simulink model "Demo_MinSegNano_V3_20b"  (R2020b)
settings: Solver=FixedStepDiscrete  StartTime=0.0  StopTime=inf  FixedStep=.03  RelTol=1e-3  EnableMultiTasking=on
undefined symbols (not defined in the file): TS
libraries: arduinolib x6, RASPlib x6, MinSegLibrary_MinSegNano x4, svdutilitieslib x4
settings Model: SILPILModeSetting=veronly  ExtModeTrigDuration=2  Creator=Alec  LastModifiedBy=hurstj
settings DataIOCC: LimitDataPoints=on  SaveFormat=Array  ReturnWorkspaceOutputs=off
settings OptimizationCC: EnhancedBackFolding=on  PassReuseOutputArgsAs=Individual arguments  ExpressionDepthLimit=2147483647  ZeroExternalMemoryAtStartup=off  ZeroInternalMemoryAtStartup=off  MaxStackSize=64  OptimizeBlockOrder=speed  DifferentSizesBufferReuse=on  OptimizationCustomize=off  EfficientTunableParamExpr=on
settings DebuggingCC: UnderspecifiedInitializationDetection=Classic  MergeDetectMultiDrivingBlocksExec=none  ParameterTunabilityLossMsg=error  StateNameClashWarn=warning  SFUnexpectedBacktrackingDiag=warning  SFNoUnconditionalDefaultTransitionDiag=warning  SFExecutionAtInitializationDiag=none  ArithmeticOperatorsInVariantConditions=warning
settings HardwareCC: ProdBitPerInt=16  ProdBitPerPointer=16  ProdBitPerSizeT=16  ProdBitPerPtrDiffT=16  ProdLargestAtomicFloat=None  ProdWordSize=8  ProdHWDeviceType=Atmel->AVR  UseEmbeddedCoderFeatures=off  UseSimulinkCoderFeatures=off
settings ModelReferenceCC: PropagateSignalLabelsOutOfModel=off
settings SFSimCC: SimUseLocalCustomCode=off  MATLABDynamicMemAlloc=off  CustomCodeUndefinedFunction=UseInterfaceOnly
settings RTWCC: Description=Embedded Coder  SystemTargetFile=ert.tlc  HardwareBoard=Arduino Nano 3.0  TemplateMakefile=ert_default_tmf  RTWVerbose=off  RTWUseLocalCustomCode=off  Toolchain=Arduino AVR  BuildConfiguration=Faster Runs
settings CodeAppCC: ForceParamTrailComments=on  IgnoreCustomStorageClasses=off  OperatorAnnotations=on  SimulinkDataObjDesc=on  SFDataObjDesc=on  CustomSymbolStrType=$N$R$M  InsertBlockDesc=on  InternalIdentifier=Classic
settings ERTTargetCC: SupportContinuousTime=on  SupportNonInlinedSFcns=on  SupportVariableSizeSignals=on  ExtModeStaticAllocSize=250
settings ConfigComp: CovMetricSettings=dw  CovSaveCumulativeToWorkspaceVar=on  CovSaveSingleToWorkspaceVar=on  CovExternalEMLEnable=off

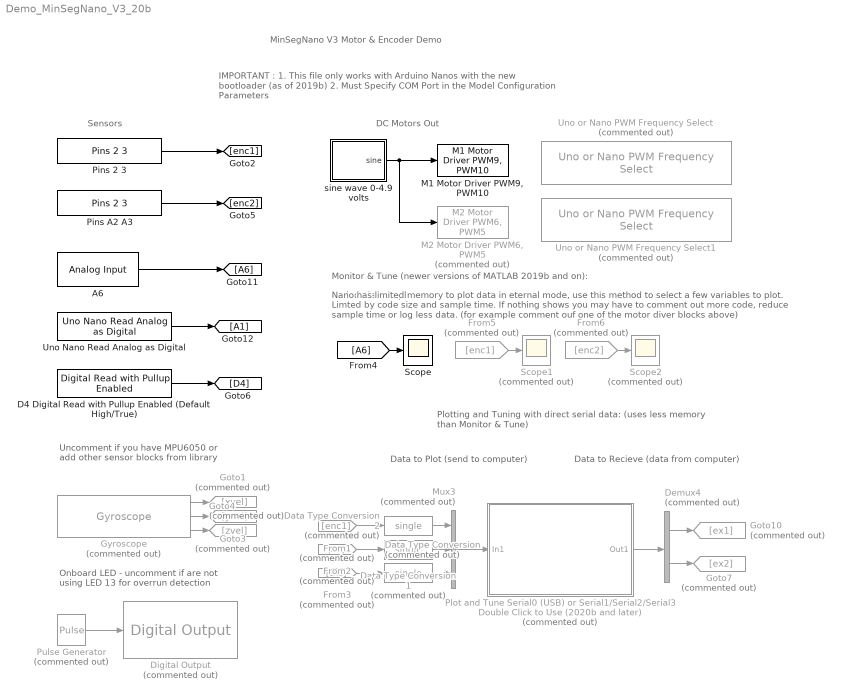
== system Demo_MinSegNano_V3_20b ==
  note: Onboard LED - uncomment if are not
      | using LED 13 for overrun detection
  note: Uncomment if you have MPU6050 or
      | add other sensor blocks from library
  note: Plotting and Tuning with direct serial data:
      | (uses less memory than Monitor & Tune)
  note: DC Motors Out
  note: Sensors
  note: MinSegNano V3 Motor & Encoder Demo
  note: IMPORTANT :
      | 1. This file only works with Arduino Nanos with the new bootloader (as of 2019b)
      | 2. Must Specify COM Port in the Model Configuration Parameters
  note: Monitor & Tune (newer versions of MATLAB 2019b and on):
  note: select data to plot
  note: Nano has limited memory to plot data in eternal mode, use this method to select a few variables to plot. Limted by code size and sample time. If nothing shows you may have to comment out more code, reduce sample time or log less data. (for example comment ouf one of the motor diver blocks above)
  note: Data to Plot
      | (send to computer)
  note: Data to Recieve
      | (data from computer)
  A6 : arduinolib/Analog Input  pinNumber=6  ReadResultsOnly=off  ConversionTriggerSource=Software  ExternalTriggerType=uint32( 0 )  OutputDataType=uint16  EnableConversionCompleteNotify=off  EnableOuputStatus=off  SampleTime=-1  blockPlatform=arduino
  D4 Digital Read with Pullup Enabled (Default High/True) : RASPlib/Digital Read with Pullup Enabled  Pin=4
      settings: SourceProductName=Rensselaer Arduino Support Package
  Data Type Conversion : DataTypeConversion  Commented=on  OutDataTypeStr=single
  Data Type Conversion1 : DataTypeConversion  Commented=on  OutDataTypeStr=single
  Data Type Conversion2 : DataTypeConversion  Commented=on  OutDataTypeStr=single
  Demux4 : Demux  Commented=on  Outputs=2
  Digital Output : arduinolib/Digital Output  Commented=on  pinNumber=13  Direction=output  blockPlatform=arduino
  From1 : From  Commented=on  GotoTag=enc1
  From2 : From  Commented=on  GotoTag=A6
  From3 : From  Commented=on  GotoTag=ex1
  From5 : From  Commented=on  GotoTag=enc1
  From6 : From  Commented=on  GotoTag=enc2
  Goto1 : Goto  Commented=on  GotoTag=xvel
  Goto10 : Goto  Commented=on  GotoTag=ex1
  Goto3 : Goto  Commented=on  GotoTag=yvel
  Goto4 : Goto  Commented=on  GotoTag=zvel
  Goto7 : Goto  Commented=on  GotoTag=ex2
  Gyroscope : RASPlib/Gyroscope  Commented=on  DLPFmode=0
      settings: SourceProductName=Rensselaer Arduino Support Package
  "M1 Motor Driver PWM9, PWM10" : MinSegLibrary_MinSegNano/M1 Motor Driver PWM9, PWM10  Vsupply=4.9  Voffset=0
      settings: SourceProductName=Rensselaer Arduino Support Package
  "M2 Motor Driver PWM6, PWM5" : MinSegLibrary_MinSegNano/M2 Motor Driver PWM6, PWM5  Commented=on  Vsupply=4.9  Voffset=0
      settings: SourceProductName=Rensselaer Arduino Support Package
  Mux3 : Mux  Commented=on  Inputs=3
  Pins 2 3 : MinSegLibrary_MinSegNano/Pins 2 3  Encoder=0  PinA=2  PinB=3
      settings: SourceProductName=Rensselaer Arduino Support Package
  Pins A2 A3 : MinSegLibrary_MinSegNano/Pins 2 3  Encoder=4  PinA=16  PinB=17
      settings: SourceProductName=Rensselaer Arduino Support Package
  Plot and Tune Serial0 (USB) or Serial1/Serial2/Serial3 Double Click to Use (2020b and later) : Subsystem  Commented=on  mask{COMport=23, Ard_Serial=0, ConnectText=<<<<<  CONNECTED  >>>>>><<<<<  CONNECTED  >>>>>><<<<<  CONNECTED  >>>>>><<<<<  CONNECTED  >>>>>>, NData=2, Data0=[1.2 3.4], DSend=[6.7 8.9]*30, Ncx=3, NumSamples=500, Parameter10=10, Parameter12=10, Parameter13=}
      mask prompts: COMport "COM Port: (device manager)"; Ard_Serial "Arduino Serial: (0 - 3)"; NData "#  Variables:"; Data0 "Initial Values:"; DSend "Data to Send:"; Ncx "# Variables:"; NumSamples "# Samples:"; Parameter10 "OnSettingChange"; Parameter12 "OnSettingChange 2"; Parameter13 "MSM9V:  [4.8341    0.2684    0.03    0.2 0 0]*0"
      mask Callback DSend: evalin('base','if(exist(''COMdevice'')),write(COMdevice,str2num(get_param(gcb,''Dsend'')),"single"),end')
      mask Callback Parameter10: set_param(gcb,'Parameter10','10')
      mask Callback Parameter12: set_param(gcb,'Parameter12','10')
      mask DialogControl DescGroupVar Prompt: Send data to/from computer to COM device.
      mask DialogControl Control9 Prompt: Connect to COM device (Microcontroller or BT).  Can press TAB to send data in the Data to Send dialog box.  Arduino Serial 0 is USB
      mask DialogControl Control3 Prompt: Connect to COM port
      mask DialogControl Control3 Callback:
      | if(evalin('base','exist(''COMdevice'')')),
      |     disp('COM port already connected');
      | else
      |    evalin('base','COMdevice=serialport([''COM'' get_param(gcb,''COMport'')],115200)')
      | end
      | set_param(gcb,'Parameter10','1')
      mask DialogControl Control6 Prompt: Disconnect COM port
      mask DialogControl Control6 Callback:
      | evalin('base','if(exist(''COMdevice'')), disp(''Closing COM port''),clear(''COMdevice''),end')
      | set_param(gcb,'Parameter10','0')
      mask DialogControl ParameterGroupVar Prompt: Tune/Recieve - Properties of Data from Computer to Microcontroller (single data type only):
      mask DialogControl Control2 Prompt: Click to Send Data
      mask DialogControl Control2 Callback:
      | %evalin('base','write(COMdevice,30,"single")')
      | evalin('base','write(COMdevice,str2num(get_param(gcb,''Dsend'')),"single")')
      mask DialogControl Container7 Prompt: Plot/Save - Properties of Data from Microntroller to Plot/Save (single data type only)
      mask DialogControl Control7 Prompt: Click to Plot Data
      mask DialogControl Control7 Callback:
      | evalin('base','if(exist(''COMdevice'')), disp(''COM port open''),else, disp(''Opening COM Port''),end')
      | set_param(gcb,'Parameter12','10') % force mask draw
      | SerialPlot_20b_Timer(['COM' get_param(gcb,'COMport')], 'single', str2num(get_param(gcb,'NumSamples')), 115200,str2num(get_param(gcb,'Ncx')))
      | set_param(gcb,'Parameter12','11') % force mask draw
      mask DialogControl Control12 Prompt: [19 0.7 0 .19]
      mask Display:
      | text(15,75,'Serial Connect Tune')
      | text(45,60,'and Plot')
      | text(35,36,'Serial Status:')
      | 
      | if(evalin('base','exist(''COMdevice'')'))
      | 
      |     patch([0 0 300 300], [0 300 300 0],[0 1 0])
      |     text(15,75,'Serial Connect Tune')
      |     text(45,60,'and Plot')
      |     text(35,36,'Serial Status:')
      |     text(0,16,'<<<  CONNECTED  >>>>')
      |     %set_param(gcb,'ConnectText','<<<<<  CONNECTED  >>>>>><<<<<  CONNECTED  >>>>>><<<<<  CONNECTED  >>>>>><<<<<  CONNECTED  >>>>>>')
      | 
      | else
      |     text(4,16,'- - - - disconnected - - - -')
      |     %set_param(gcb,'ConnectText','- - - - - - disconnected - - - - - -- - - - - - disconnected - - - - - -- - - - - - disconnected - - - - - -- - - - - - disconnected - - - - - -- - - - - - disconnected - - - - - -')
      | end
  Pulse Generator : DiscretePulseGenerator  Commented=on  PulseType=Time based  Period=10  PulseWidth=5
  Scope : Scope
  Scope1 : Scope  Commented=on
  Scope2 : Scope  Commented=on
  Uno Nano Read Analog as Digital : RASPlib/Uno Nano Read Analog as Digital  Pin=1
      settings: SourceProductName=Rensselaer Arduino Support Package
  Uno or Nano PWM Frequency Select : RASPlib/Uno or Nano PWM Frequency Select  Commented=on  Frequency=490Hz (Timer 0: 976Hz)  Timer=1 - pins 9, 10
      settings: SourceProductName=Rensselaer Arduino Support Package
  Uno or Nano PWM Frequency Select1 : RASPlib/Uno or Nano PWM Frequency Select  Commented=on  Frequency=490Hz (Timer 0: 976Hz)  Timer=0 - pins 5, 6
      settings: SourceProductName=Rensselaer Arduino Support Package
  sine wave 0-4.9 volts : Subsystem
  wires:
  A6/1 -> [A6]
  Uno Nano Read Analog as Digital/1 -> [A1]
  Gyroscope/1 -> Goto1/1
  Pulse Generator/1 -> Digital Output/1
  Gyroscope/2 -> Goto3/1
  Gyroscope/3 -> Goto4/1
  Pins 2 3/1 -> [enc1]
  Pins A2 A3/1 -> [enc2]
  D4 Digital Read with Pullup Enabled (Default High/True)/1 -> [D4]
  sine wave 0-4.9 volts/1(sine) -> "M2 Motor Driver PWM6, PWM5"/1, "M1 Motor Driver PWM9, PWM10"/1
  [A6] -> Scope/1
  From5/1 -> Scope1/1
  From6/1 -> Scope2/1
  Mux3/1 -> Plot and Tune Serial0 (USB) or Serial1/Serial2/Serial3 Double Click to Use (2020b and later)/1(In1)
  Plot and Tune Serial0 (USB) or Serial1/Serial2/Serial3 Double Click to Use (2020b and later)/1(Out1) -> Demux4/1
  Demux4/1 -> Goto10/1
  Demux4/2 -> Goto7/1
  Data Type Conversion/1 -> Mux3/3
  Data Type Conversion1/1 -> Mux3/2
  Data Type Conversion2/1 -> Mux3/1
  From1/1 -> Data Type Conversion2/1
  From2/1 -> Data Type Conversion1/1
  From3/1 -> Data Type Conversion/1

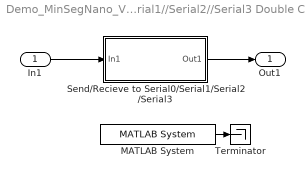
== system Demo_MinSegNano_V3_20b/Plot and Tune Serial0 (USB) or Serial1//Serial2//Serial3 Double Click to Use (2020b and later) ==
  In1 : Inport
  MATLAB System : RASPlib/Double Click to Plot Serial Data/MATLAB System  is_post_2015a=~verLessThan( 'matlab', '8.6' )
      settings: SourceProductName=Rensselaer Arduino Support Package
  Send/Recieve to Serial0/Serial1/Serial2/Serial3 : Subsystem  Variant=on
  Terminator : Terminator
  Out1 : Outport
  wires:
  Send/Recieve to Serial0/Serial1/Serial2/Serial3/1(Out1) -> Out1/1
  In1/1 -> Send/Recieve to Serial0/Serial1/Serial2/Serial3/1(In1)
  MATLAB System/1 -> Terminator/1

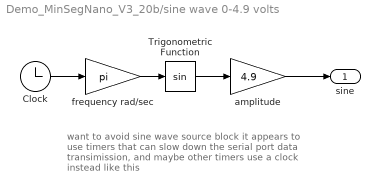
== system Demo_MinSegNano_V3_20b/sine wave 0-4.9 volts ==
  note: want to avoid sine wave source block
      | it appears to use timers that can slow down the
      | serial port data transimission, and maybe
      | other timers
      |
      | use a clock instead like this
  Clock : Clock
  Trigonometric Function : Trigonometry
  amplitude : Gain  Gain=4.9
  frequency rad/sec : Gain  Gain=pi
  sine : Outport
  wires:
  amplitude/1 -> sine/1
  frequency rad/sec/1 -> Trigonometric Function/1
  Trigonometric Function/1 -> amplitude/1
  Clock/1 -> frequency rad/sec/1

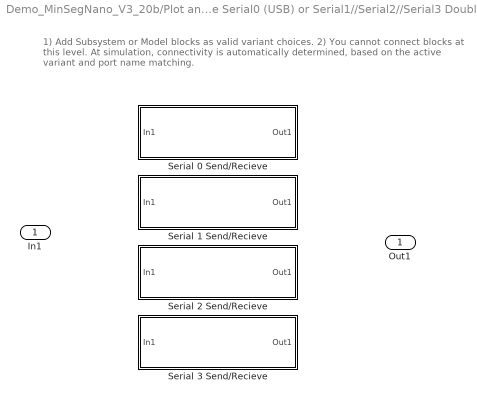
== system Demo_MinSegNano_V3_20b/Plot and Tune Serial0 (USB) or Serial1//Serial2//Serial3 Double Click to Use (2020b and later)/Send//Recieve to Serial0//Serial1//Serial2//Serial3 ==
  note: 1) Add Subsystem or Model blocks as valid variant choices.
      | 2) You cannot connect blocks at this level. At simulation, connectivity is automatically
      | determined, based on the active variant and port name matching.
  In1 : Inport
  Serial 0 Send/Recieve : Subsystem  VariantControl=Ard_Serial==0
  Serial 1 Send/Recieve : Subsystem  VariantControl=Ard_Serial==1
  Serial 2 Send/Recieve : Subsystem  VariantControl=Ard_Serial==2
  Serial 3 Send/Recieve : Subsystem  VariantControl=Ard_Serial==3
  Out1 : Outport

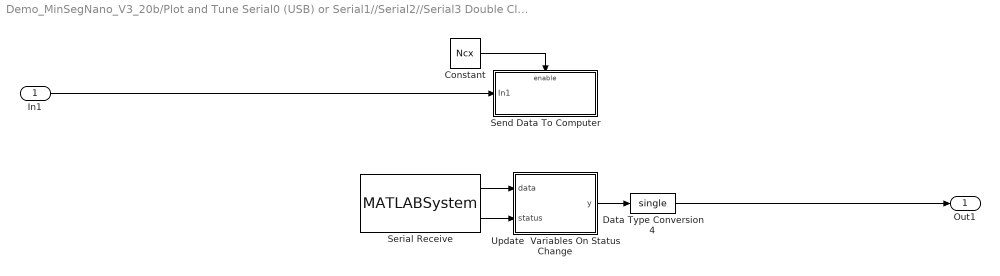
== system Demo_MinSegNano_V3_20b/Plot and Tune Serial0 (USB) or Serial1//Serial2//Serial3 Double Click to Use (2020b and later)/Send//Recieve to Serial0//Serial1//Serial2//Serial3/Serial 0 Send//Recieve ==
  In1 : Inport
  Constant : Constant  Value=Ncx
  Data Type Conversion4 : DataTypeConversion  OutDataTypeStr=single
  Send Data To Computer : Subsystem  TreatAsAtomicUnit=on
  Serial Receive : MATLABSystem  InitFcn=|  System=codertarget.arduinobase.internal.arduino_SerialRead  isARMArch=off  portNumber=portNumber  SampleTime=SampleTime  DataType=double  Datalength=Datalength  Protocol=0  mask(Arduino Serial Receive){isARMArch=off, portNumber=0, DataType=double, Datalength=NData, SampleTime=str2num(get_param(bdroot,'FixedStep')), showOutStatus=on, blockPlatform=arduino}
      | %codertarget.arduinobase.blocks.arduinoBlockInitFcnCallback(gcbh);
      | %codertarget.arduinobase.blocks.registerSerialBlock(gcbh);
      mask prompts: isARMArch "Is ARM Architecture"; portNumber "Port number:"; DataType "Data type:"; Datalength "Data length:"; SampleTime "Sample time:"; showOutStatus "Output receiving status"; blockPlatform "Block platform:"
      mask help:
      | Receive an [Nx1] array of data on the specified serial port and write it to the Data block output.When data is not available, write 0 to the Data block output.
      |
      | The Status port outputs 0 when the length of data received is less than the Data length specified. Otherwise, it emits 1.
      |
      | Use the Data length parameter to specify the number of data bytes  to receive.
      mask init:
      | codertarget.arduinobase.blocks.arduinoSerialReadCallback('MaskInitialization');
      mask Help: eval('codertarget.internal.helpView(''arduinoert'', ''arduinolibarduinoserialreceive'')')
      mask TypeOptions isARMArch: isARMArch
      mask Callback isARMArch: codertarget.arduinobase.blocks.arduinoSerialReadCallback('isARMArch');
      mask TypeOptions portNumber: portNumber
      mask TypeOptions DataType: DataType
      mask TypeOptions Datalength: Datalength
      mask TypeOptions SampleTime: SampleTime
      mask DialogControl Control2 Prompt: View pin map
      mask DialogControl Control2 Callback:
      | file = [codertarget.arduinobase.internal.getBaseSpPkgRootDir filesep 'blocks' filesep 'mex' filesep 'arduinoPinMapping.html'];
      | web(file)
      mask Display:
      | pic=imread('serial.png');image(pic,[0.28 0.18 0.45 0.65]);text(0.5, 0.15, 'Port 0', 'horizontalAlignment', 'center');
      | color('blue');
      | text(0.55, 0.87, 'ARDUINO', 'horizontalAlignment', 'left');
      | color('black');
      | port_label('output', 1, 'Data');
      | port_label('output', 2, 'Status');
  Update  Variables On Status Change : Subsystem
  Out1 : Outport
  wires:
  Data Type Conversion4/1 -> Out1/1
  Serial Receive/1 -> Update  Variables On Status Change/1(data)
  Serial Receive/2 -> Update  Variables On Status Change/2(status)
  Constant/1 -> Send Data To Computer/Enable
  In1/1 -> Send Data To Computer/1(In1)
  Update  Variables On Status Change/1(y) -> Data Type Conversion4/1

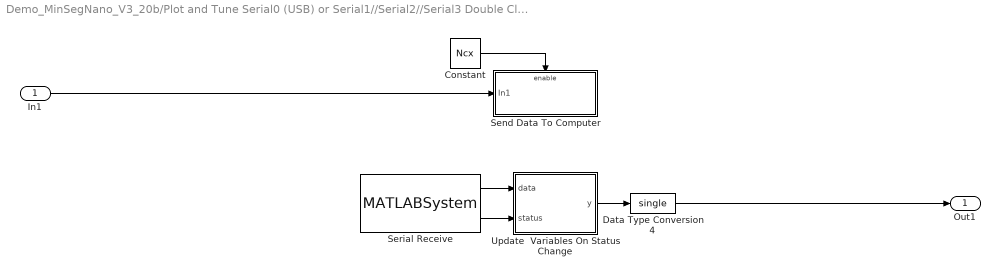
== system Demo_MinSegNano_V3_20b/Plot and Tune Serial0 (USB) or Serial1//Serial2//Serial3 Double Click to Use (2020b and later)/Send//Recieve to Serial0//Serial1//Serial2//Serial3/Serial 1 Send//Recieve ==
  In1 : Inport
  Constant : Constant  Value=Ncx
  Data Type Conversion4 : DataTypeConversion  OutDataTypeStr=single
  Send Data To Computer : Subsystem  TreatAsAtomicUnit=on
  Serial Receive : MATLABSystem  InitFcn=|  System=codertarget.arduinobase.internal.arduino_SerialRead  isARMArch=off  portNumber=portNumber  SampleTime=SampleTime  DataType=double  Datalength=Datalength  Protocol=0  mask(Arduino Serial Receive){isARMArch=off, portNumber=1, DataType=double, Datalength=NData, SampleTime=TS, showOutStatus=on, blockPlatform=arduino}
      | %codertarget.arduinobase.blocks.arduinoBlockInitFcnCallback(gcbh);
      | %codertarget.arduinobase.blocks.registerSerialBlock(gcbh);
      mask prompts: isARMArch "Is ARM Architecture"; portNumber "Port number:"; DataType "Data type:"; Datalength "Data length:"; SampleTime "Sample time:"; showOutStatus "Output receiving status"; blockPlatform "Block platform:"
      mask help:
      | Receive an [Nx1] array of data on the specified serial port and write it to the Data block output.When data is not available, write 0 to the Data block output.
      |
      | The Status port outputs 0 when the length of data received is less than the Data length specified. Otherwise, it emits 1.
      |
      | Use the Data length parameter to specify the number of data bytes  to receive.
      mask init:
      | codertarget.arduinobase.blocks.arduinoSerialReadCallback('MaskInitialization');
      mask Help: eval('codertarget.internal.helpView(''arduinoert'', ''arduinolibarduinoserialreceive'')')
      mask TypeOptions isARMArch: isARMArch
      mask Callback isARMArch: codertarget.arduinobase.blocks.arduinoSerialReadCallback('isARMArch');
      mask TypeOptions portNumber: portNumber
      mask TypeOptions DataType: DataType
      mask TypeOptions Datalength: Datalength
      mask TypeOptions SampleTime: SampleTime
      mask DialogControl Control2 Prompt: View pin map
      mask DialogControl Control2 Callback:
      | file = [codertarget.arduinobase.internal.getBaseSpPkgRootDir filesep 'blocks' filesep 'mex' filesep 'arduinoPinMapping.html'];
      | web(file)
      mask Display:
      | pic=imread('serial.png');image(pic,[0.28 0.18 0.45 0.65]);text(0.5, 0.15, 'Port 1', 'horizontalAlignment', 'center');
      | color('blue');
      | text(0.55, 0.87, 'ARDUINO', 'horizontalAlignment', 'left');
      | color('black');
      | port_label('output', 1, 'Data');
      | port_label('output', 2, 'Status');
  Update  Variables On Status Change : Subsystem
  Out1 : Outport
  wires:
  Update  Variables On Status Change/1(y) -> Data Type Conversion4/1
  In1/1 -> Send Data To Computer/1(In1)
  Constant/1 -> Send Data To Computer/Enable
  Serial Receive/2 -> Update  Variables On Status Change/2(status)
  Serial Receive/1 -> Update  Variables On Status Change/1(data)
  Data Type Conversion4/1 -> Out1/1

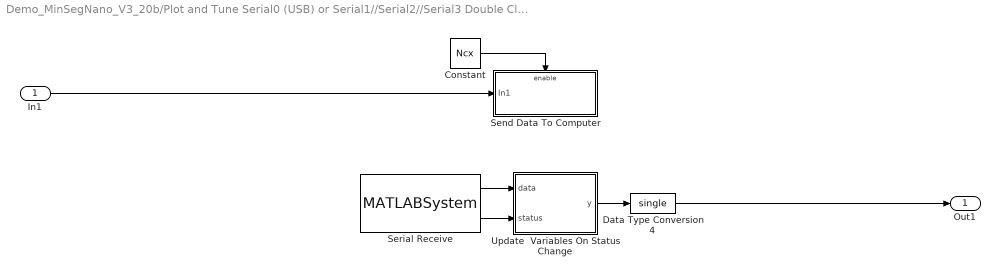
== system Demo_MinSegNano_V3_20b/Plot and Tune Serial0 (USB) or Serial1//Serial2//Serial3 Double Click to Use (2020b and later)/Send//Recieve to Serial0//Serial1//Serial2//Serial3/Serial 2 Send//Recieve ==
  In1 : Inport
  Constant : Constant  Value=Ncx
  Data Type Conversion4 : DataTypeConversion  OutDataTypeStr=single
  Send Data To Computer : Subsystem  TreatAsAtomicUnit=on
  Serial Receive : MATLABSystem  InitFcn=|  System=codertarget.arduinobase.internal.arduino_SerialRead  isARMArch=off  portNumber=portNumber  SampleTime=SampleTime  DataType=double  Datalength=Datalength  Protocol=0  mask(Arduino Serial Receive){isARMArch=off, portNumber=2, DataType=double, Datalength=NData, SampleTime=TS, showOutStatus=on, blockPlatform=arduino}
      | %codertarget.arduinobase.blocks.arduinoBlockInitFcnCallback(gcbh);
      | %codertarget.arduinobase.blocks.registerSerialBlock(gcbh);
      mask prompts: isARMArch "Is ARM Architecture"; portNumber "Port number:"; DataType "Data type:"; Datalength "Data length:"; SampleTime "Sample time:"; showOutStatus "Output receiving status"; blockPlatform "Block platform:"
      mask help:
      | Receive an [Nx1] array of data on the specified serial port and write it to the Data block output.When data is not available, write 0 to the Data block output.
      |
      | The Status port outputs 0 when the length of data received is less than the Data length specified. Otherwise, it emits 1.
      |
      | Use the Data length parameter to specify the number of data bytes  to receive.
      mask init:
      | codertarget.arduinobase.blocks.arduinoSerialReadCallback('MaskInitialization');
      mask Help: eval('codertarget.internal.helpView(''arduinoert'', ''arduinolibarduinoserialreceive'')')
      mask TypeOptions isARMArch: isARMArch
      mask Callback isARMArch: codertarget.arduinobase.blocks.arduinoSerialReadCallback('isARMArch');
      mask TypeOptions portNumber: portNumber
      mask TypeOptions DataType: DataType
      mask TypeOptions Datalength: Datalength
      mask TypeOptions SampleTime: SampleTime
      mask DialogControl Control2 Prompt: View pin map
      mask DialogControl Control2 Callback:
      | file = [codertarget.arduinobase.internal.getBaseSpPkgRootDir filesep 'blocks' filesep 'mex' filesep 'arduinoPinMapping.html'];
      | web(file)
      mask Display:
      | pic=imread('serial.png');image(pic,[0.28 0.18 0.45 0.65]);text(0.5, 0.15, 'Port 2', 'horizontalAlignment', 'center');
      | color('blue');
      | text(0.55, 0.87, 'ARDUINO', 'horizontalAlignment', 'left');
      | color('black');
      | port_label('output', 1, 'Data');
      | port_label('output', 2, 'Status');
  Update  Variables On Status Change : Subsystem
  Out1 : Outport
  wires:
  Data Type Conversion4/1 -> Out1/1
  Serial Receive/1 -> Update  Variables On Status Change/1(data)
  Serial Receive/2 -> Update  Variables On Status Change/2(status)
  Constant/1 -> Send Data To Computer/Enable
  In1/1 -> Send Data To Computer/1(In1)
  Update  Variables On Status Change/1(y) -> Data Type Conversion4/1

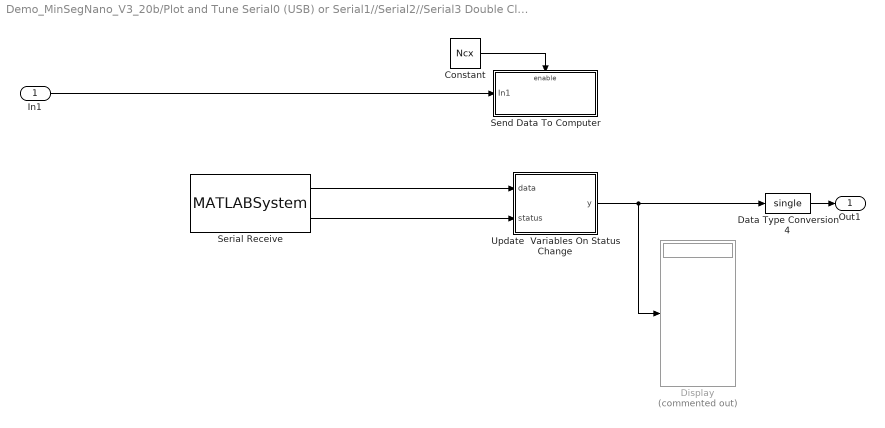
== system Demo_MinSegNano_V3_20b/Plot and Tune Serial0 (USB) or Serial1//Serial2//Serial3 Double Click to Use (2020b and later)/Send//Recieve to Serial0//Serial1//Serial2//Serial3/Serial 3 Send//Recieve ==
  In1 : Inport
  Constant : Constant  Value=Ncx
  Data Type Conversion4 : DataTypeConversion  OutDataTypeStr=single
  Display : Display  Commented=on
  Send Data To Computer : Subsystem  TreatAsAtomicUnit=on
  Serial Receive : MATLABSystem  InitFcn=|  System=codertarget.arduinobase.internal.arduino_SerialRead  isARMArch=off  portNumber=portNumber  SampleTime=SampleTime  DataType=double  Datalength=Datalength  Protocol=0  mask(Arduino Serial Receive){isARMArch=off, portNumber=3, DataType=double, Datalength=NData, SampleTime=TS, showOutStatus=on, blockPlatform=arduino}
      | %codertarget.arduinobase.blocks.arduinoBlockInitFcnCallback(gcbh);
      | %codertarget.arduinobase.blocks.registerSerialBlock(gcbh);
      mask prompts: isARMArch "Is ARM Architecture"; portNumber "Port number:"; DataType "Data type:"; Datalength "Data length:"; SampleTime "Sample time:"; showOutStatus "Output receiving status"; blockPlatform "Block platform:"
      mask help:
      | Receive an [Nx1] array of data on the specified serial port and write it to the Data block output.When data is not available, write 0 to the Data block output.
      |
      | The Status port outputs 0 when the length of data received is less than the Data length specified. Otherwise, it emits 1.
      |
      | Use the Data length parameter to specify the number of data bytes  to receive.
      mask init:
      | codertarget.arduinobase.blocks.arduinoSerialReadCallback('MaskInitialization');
      mask Help: eval('codertarget.internal.helpView(''arduinoert'', ''arduinolibarduinoserialreceive'')')
      mask TypeOptions isARMArch: isARMArch
      mask Callback isARMArch: codertarget.arduinobase.blocks.arduinoSerialReadCallback('isARMArch');
      mask TypeOptions portNumber: portNumber
      mask TypeOptions DataType: DataType
      mask TypeOptions Datalength: Datalength
      mask TypeOptions SampleTime: SampleTime
      mask DialogControl Control2 Prompt: View pin map
      mask DialogControl Control2 Callback:
      | file = [codertarget.arduinobase.internal.getBaseSpPkgRootDir filesep 'blocks' filesep 'mex' filesep 'arduinoPinMapping.html'];
      | web(file)
      mask Display:
      | pic=imread('serial.png');image(pic,[0.28 0.18 0.45 0.65]);text(0.5, 0.15, 'Port 3', 'horizontalAlignment', 'center');
      | color('blue');
      | text(0.55, 0.87, 'ARDUINO', 'horizontalAlignment', 'left');
      | color('black');
      | port_label('output', 1, 'Data');
      | port_label('output', 2, 'Status');
  Update  Variables On Status Change : Subsystem
  Out1 : Outport
  wires:
  In1/1 -> Send Data To Computer/1(In1)
  Constant/1 -> Send Data To Computer/Enable
  Serial Receive/2 -> Update  Variables On Status Change/2(status)
  Data Type Conversion4/1 -> Out1/1
  Serial Receive/1 -> Update  Variables On Status Change/1(data)
  Update  Variables On Status Change/1(y) -> Display/1, Data Type Conversion4/1

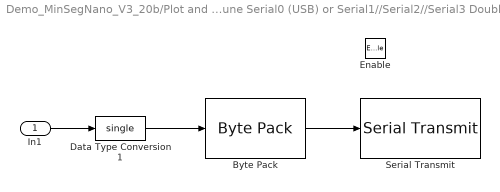
== system Demo_MinSegNano_V3_20b/Plot and Tune Serial0 (USB) or Serial1//Serial2//Serial3 Double Click to Use (2020b and later)/Send//Recieve to Serial0//Serial1//Serial2//Serial3/Serial 0 Send//Recieve/Send Data To Computer ==
  In1 : Inport
  Enable : EnablePort
  Byte Pack : svdutilitieslib/Byte Pack  maskPackedDataType=uint8  datatypes={'single'}  byteAlign=1  blockPlatform=arduinoert
      settings: SourceProductBaseCode=ANDROID,ARDUINO,ML_ARDUINO,ECCORTEXA,ECCORTEXR,SC_BEAGLEBONE_BLUE,EC_FREEDOM_BOARD,EC_FRDM_K64F,INTEL_BLOCKSET,JETSONCPU,MICROBIT,NUCLEO,NVIDIA,PX4AUTOPILOTS,RASPPIIO,STMICRODIS,TIC2000,XILINX_BLOCKSET
  Data Type Conversion1 : DataTypeConversion  OutDataTypeStr=single
  Serial Transmit : arduinolib/Serial Transmit  portNumber=0  sendmode=write  sendformat=Decimal  floatprecision=2  blockPlatform=arduino
  wires:
  In1/1 -> Data Type Conversion1/1
  Data Type Conversion1/1 -> Byte Pack/1
  Byte Pack/1 -> Serial Transmit/1

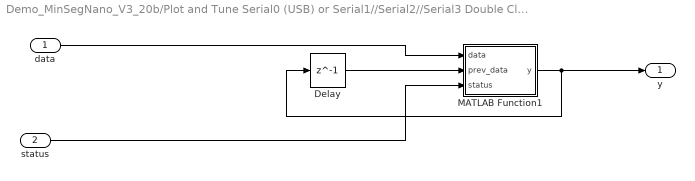
== system Demo_MinSegNano_V3_20b/Plot and Tune Serial0 (USB) or Serial1//Serial2//Serial3 Double Click to Use (2020b and later)/Send//Recieve to Serial0//Serial1//Serial2//Serial3/Serial 0 Send//Recieve/Update  Variables On Status Change ==
  data : Inport
  status : Inport  Port=2
  Delay : Delay  DelayLength=1  InitialCondition=Data0
  MATLAB Function1 : MATLAB Function  TreatAsAtomicUnit=on
  y : Outport
  wires:
  status/1 -> MATLAB Function1/3(status)
  data/1 -> MATLAB Function1/1(data)
  MATLAB Function1/1(y) -> y/1, Delay/1
  Delay/1 -> MATLAB Function1/2(prev_data)

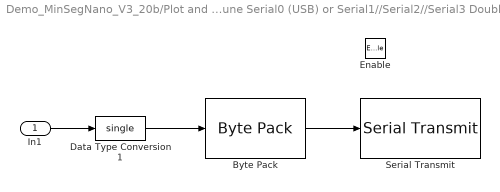
== system Demo_MinSegNano_V3_20b/Plot and Tune Serial0 (USB) or Serial1//Serial2//Serial3 Double Click to Use (2020b and later)/Send//Recieve to Serial0//Serial1//Serial2//Serial3/Serial 1 Send//Recieve/Send Data To Computer ==
  In1 : Inport
  Enable : EnablePort
  Byte Pack : svdutilitieslib/Byte Pack  maskPackedDataType=uint8  datatypes={'single'}  byteAlign=1  blockPlatform=arduinoert
      settings: SourceProductBaseCode=ANDROID,ARDUINO,ML_ARDUINO,ECCORTEXA,ECCORTEXR,SC_BEAGLEBONE_BLUE,EC_FREEDOM_BOARD,EC_FRDM_K64F,INTEL_BLOCKSET,JETSONCPU,MICROBIT,NUCLEO,NVIDIA,PX4AUTOPILOTS,RASPPIIO,STMICRODIS,TIC2000,XILINX_BLOCKSET
  Data Type Conversion1 : DataTypeConversion  OutDataTypeStr=single
  Serial Transmit : arduinolib/Serial Transmit  portNumber=1  sendmode=write  sendformat=Decimal  floatprecision=2  blockPlatform=arduino
  wires:
  Byte Pack/1 -> Serial Transmit/1
  Data Type Conversion1/1 -> Byte Pack/1
  In1/1 -> Data Type Conversion1/1

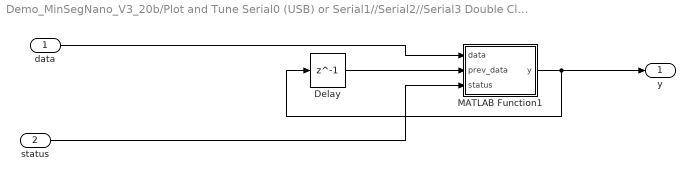
== system Demo_MinSegNano_V3_20b/Plot and Tune Serial0 (USB) or Serial1//Serial2//Serial3 Double Click to Use (2020b and later)/Send//Recieve to Serial0//Serial1//Serial2//Serial3/Serial 1 Send//Recieve/Update  Variables On Status Change ==
  data : Inport
  status : Inport  Port=2
  Delay : Delay  DelayLength=1  InitialCondition=Data0  SampleTime=TS
  MATLAB Function1 : MATLAB Function  TreatAsAtomicUnit=on
  y : Outport
  wires:
  Delay/1 -> MATLAB Function1/2(prev_data)
  MATLAB Function1/1(y) -> Delay/1, y/1
  data/1 -> MATLAB Function1/1(data)
  status/1 -> MATLAB Function1/3(status)

== system Demo_MinSegNano_V3_20b/Plot and Tune Serial0 (USB) or Serial1//Serial2//Serial3 Double Click to Use (2020b and later)/Send//Recieve to Serial0//Serial1//Serial2//Serial3/Serial 2 Send//Recieve/Send Data To Computer ==
  In1 : Inport
  Enable : EnablePort
  Byte Pack : svdutilitieslib/Byte Pack  maskPackedDataType=uint8  datatypes={'single'}  byteAlign=1  blockPlatform=arduinoert
      settings: SourceProductBaseCode=ANDROID,ARDUINO,ML_ARDUINO,ECCORTEXA,ECCORTEXR,SC_BEAGLEBONE_BLUE,EC_FREEDOM_BOARD,EC_FRDM_K64F,INTEL_BLOCKSET,JETSONCPU,MICROBIT,NUCLEO,NVIDIA,PX4AUTOPILOTS,RASPPIIO,STMICRODIS,TIC2000,XILINX_BLOCKSET
  Data Type Conversion1 : DataTypeConversion  OutDataTypeStr=single
  Serial Transmit : arduinolib/Serial Transmit  portNumber=2  sendmode=write  sendformat=Decimal  floatprecision=2  blockPlatform=arduino
  wires:
  In1/1 -> Data Type Conversion1/1
  Data Type Conversion1/1 -> Byte Pack/1
  Byte Pack/1 -> Serial Transmit/1

== system Demo_MinSegNano_V3_20b/Plot and Tune Serial0 (USB) or Serial1//Serial2//Serial3 Double Click to Use (2020b and later)/Send//Recieve to Serial0//Serial1//Serial2//Serial3/Serial 2 Send//Recieve/Update  Variables On Status Change ==
  data : Inport
  status : Inport  Port=2
  Delay : Delay  DelayLength=1  InitialCondition=Data0  SampleTime=TS
  MATLAB Function1 : MATLAB Function  TreatAsAtomicUnit=on
  y : Outport
  wires:
  status/1 -> MATLAB Function1/3(status)
  data/1 -> MATLAB Function1/1(data)
  MATLAB Function1/1(y) -> y/1, Delay/1
  Delay/1 -> MATLAB Function1/2(prev_data)

== system Demo_MinSegNano_V3_20b/Plot and Tune Serial0 (USB) or Serial1//Serial2//Serial3 Double Click to Use (2020b and later)/Send//Recieve to Serial0//Serial1//Serial2//Serial3/Serial 3 Send//Recieve/Send Data To Computer ==
  In1 : Inport
  Enable : EnablePort
  Byte Pack : svdutilitieslib/Byte Pack  maskPackedDataType=uint8  datatypes={'single'}  byteAlign=1  blockPlatform=arduinoert
      settings: SourceProductBaseCode=ANDROID,ARDUINO,ML_ARDUINO,ECCORTEXA,ECCORTEXR,SC_BEAGLEBONE_BLUE,EC_FREEDOM_BOARD,EC_FRDM_K64F,INTEL_BLOCKSET,JETSONCPU,MICROBIT,NUCLEO,NVIDIA,PX4AUTOPILOTS,RASPPIIO,STMICRODIS,TIC2000,XILINX_BLOCKSET
  Data Type Conversion1 : DataTypeConversion  OutDataTypeStr=single
  Serial Transmit : arduinolib/Serial Transmit  portNumber=3  sendmode=write  sendformat=Decimal  floatprecision=2  blockPlatform=arduino
  wires:
  Byte Pack/1 -> Serial Transmit/1
  Data Type Conversion1/1 -> Byte Pack/1
  In1/1 -> Data Type Conversion1/1

== system Demo_MinSegNano_V3_20b/Plot and Tune Serial0 (USB) or Serial1//Serial2//Serial3 Double Click to Use (2020b and later)/Send//Recieve to Serial0//Serial1//Serial2//Serial3/Serial 3 Send//Recieve/Update  Variables On Status Change ==
  data : Inport
  status : Inport  Port=2
  Delay : Delay  DelayLength=1  InitialCondition=[Data0]  SampleTime=TS
  MATLAB Function1 : MATLAB Function  TreatAsAtomicUnit=on
  y : Outport
  wires:
  Delay/1 -> MATLAB Function1/2(prev_data)
  MATLAB Function1/1(y) -> Delay/1, y/1
  data/1 -> MATLAB Function1/1(data)
  status/1 -> MATLAB Function1/3(status)

== matlab function Demo_MinSegNano_V3_20b/Plot and Tune Serial0 (USB) or Serial1//Serial2//Serial3 Double Click to Use (2020b and later)/Send//Recieve to Serial0//Serial1//Serial2//Serial3/Serial 1 Send//Recieve/Update  Variables On Status Change/MATLAB Function1 ==
  data: data input; y output; prev_data input; status input
function y= fcn(data,prev_data,status)

if(status)
    y=data;
else
    y=prev_data;
end

== matlab function Demo_MinSegNano_V3_20b/Plot and Tune Serial0 (USB) or Serial1//Serial2//Serial3 Double Click to Use (2020b and later)/Send//Recieve to Serial0//Serial1//Serial2//Serial3/Serial 3 Send//Recieve/Update  Variables On Status Change/MATLAB Function1 ==
  data: data input; y output; prev_data input; status input
function y= fcn(data,prev_data,status)

if(status)
    y=data;
else
    y=prev_data;
end

== matlab function Demo_MinSegNano_V3_20b/Plot and Tune Serial0 (USB) or Serial1//Serial2//Serial3 Double Click to Use (2020b and later)/Send//Recieve to Serial0//Serial1//Serial2//Serial3/Serial 0 Send//Recieve/Update  Variables On Status Change/MATLAB Function1 ==
  data: data input; y output; prev_data input; status input
function y= fcn(data,prev_data,status)

if(status)
    y=data;
else
    y=prev_data;
end

== matlab function Demo_MinSegNano_V3_20b/Plot and Tune Serial0 (USB) or Serial1//Serial2//Serial3 Double Click to Use (2020b and later)/Send//Recieve to Serial0//Serial1//Serial2//Serial3/Serial 2 Send//Recieve/Update  Variables On Status Change/MATLAB Function1 ==
  data: data input; y output; prev_data input; status input
function y= fcn(data,prev_data,status)

if(status)
    y=data;
else
    y=prev_data;
end
